simulink model "tv_system_sqabs"  (R2021b)
settings: Solver=VariableStepAuto  StartTime=0.0  StopTime=0  RelTol=1e-3
values from neighbouring files (symbols this model uses):
  gamma1 = 0.005    [main_pixloss.m]
  gamma2 = 1/(1.05*tau2)*(1/gamma1-beta/2)    [main_pixloss.m]
  lambda = 0.012    [main_pixloss.m]
  maxIter = 500    [main_pixloss.m]
undefined symbols (not defined in the file or in its folder): cols, gray, rows
libraries: visionsources x3, visionstatistics x2
settings Model: Creator=abeshu  LastModifiedBy=shu_abe

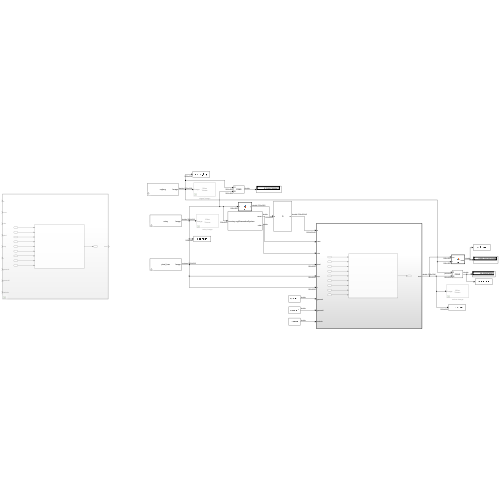
[thumbnail: Simulink's stored preview of the top-level diagram]
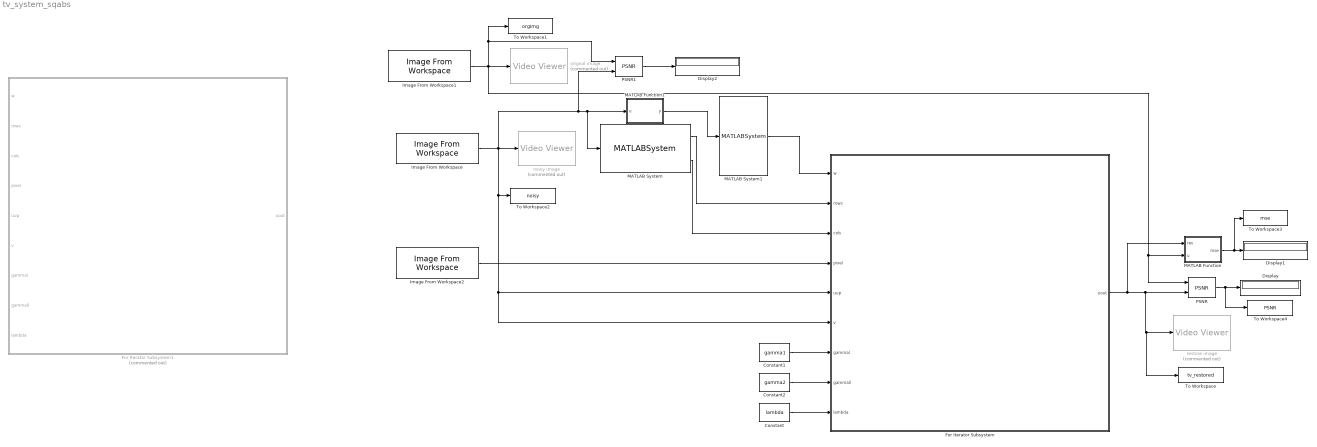
== system tv_system_sqabs ==
  Constant : Constant  Value=lambda
  Constant1 : Constant  Value=gamma1
  Constant2 : Constant  Value=gamma2
  Display : Display
  Display1 : Display
  Display2 : Display
  For Iterator Subsystem : Subsystem  TreatAsAtomicUnit=on
  For Iterator Subsystem1 : Subsystem  Commented=on  TreatAsAtomicUnit=on
  Image From Workspace : visionsources/Image From Workspace  Tag=vipblks_nd  ImageValue=noisy  Ts=inf  imagePorts=One multidimensional signal  OutPortLabels=R|G|B  ImageDataType=Inherit from 'Value'  Signed=on  WordLength=16  sdImageDataType=sfix(16)  FractionLengthMode=User-defined  FractionLength=15
      settings: SourceProductBaseCode=VP
  Image From Workspace1 : visionsources/Image From Workspace  Tag=vipblks_nd  ImageValue=orgImg  Ts=inf  imagePorts=One multidimensional signal  OutPortLabels=R|G|B  ImageDataType=Inherit from 'Value'  Signed=on  WordLength=16  sdImageDataType=sfix(16)  FractionLengthMode=User-defined  FractionLength=15
      settings: SourceProductBaseCode=VP
  Image From Workspace2 : visionsources/Image From Workspace  Tag=vipblks_nd  ImageValue=pixel_loss  Ts=inf  imagePorts=One multidimensional signal  OutPortLabels=R|G|B  ImageDataType=Inherit from 'Value'  Signed=on  WordLength=16  sdImageDataType=sfix(16)  FractionLengthMode=User-defined  FractionLength=15
      settings: SourceProductBaseCode=VP
  MATLAB Function : MATLAB Function  TreatAsAtomicUnit=on
  MATLAB Function1 : MATLAB Function  TreatAsAtomicUnit=on
  MATLAB System : MATLABSystem  System=regObsevationSystem  SimulateUsing=Code generation
      mask Type: regObsevationSystem
      mask Display:
      | disp('regObsevationSystem');
      | port_label('input',1,'imnoisy');
      | port_label('output',1,'rows');
      | port_label('output',2,'colw');
  MATLAB System1 : MATLABSystem  System=dBlockSystem  SimulateUsing=Code generation
      mask Type: dBlockSystem
      mask Display:
      | disp('D');
      | port_label('input',1,'z');
      | port_label('output',1,'w');
  PSNR : visionstatistics/PSNR
      settings: SourceProductBaseCode=VP
  PSNR1 : visionstatistics/PSNR
      settings: SourceProductBaseCode=VP
  To Workspace : ToWorkspace  VariableName=tv_restored  SaveFormat=Structure  SampleTime=-1
      settings: Save2DSignal=2-D array (concatenate along first dimension)
  To Workspace1 : ToWorkspace  VariableName=orgImg  SaveFormat=Structure  SampleTime=-1
      settings: Save2DSignal=2-D array (concatenate along first dimension)
  To Workspace2 : ToWorkspace  VariableName=noisy  SaveFormat=Structure  SampleTime=-1
      settings: Save2DSignal=2-D array (concatenate along first dimension)
  To Workspace3 : ToWorkspace  VariableName=mse  SaveFormat=Structure  SampleTime=-1
      settings: Save2DSignal=2-D array (concatenate along first dimension)
  To Workspace4 : ToWorkspace  VariableName=PSNR  SaveFormat=Structure  SampleTime=-1
      settings: Save2DSignal=2-D array (concatenate along first dimension)
  noisy image : VideoViewer  Commented=on  FigPos=[211 982 368 339]
  orignal image : VideoViewer  Commented=on  FigPos=[20 546 468 269]
  restore image : VideoViewer  Commented=on  colormapValue=gray(256)  FigPos=[260 843 480 394]
  wires:
  Image From Workspace/1 -> For Iterator Subsystem/6(v), For Iterator Subsystem/5(uup), To Workspace2/1, PSNR1/2, MATLAB System/1, MATLAB Function1/1(u), noisy image/1
  Image From Workspace1/1 -> PSNR1/1, To Workspace1/1, PSNR/1, MATLAB Function/2(u), orignal image/1
  Image From Workspace2/1 -> For Iterator Subsystem/4(pixel)
  MATLAB System/1 -> For Iterator Subsystem/2(rows)
  MATLAB System/2 -> For Iterator Subsystem/3(cols)
  MATLAB Function1/1(y) -> MATLAB System1/1
  Constant1/1 -> For Iterator Subsystem/7(gammal)
  Constant2/1 -> For Iterator Subsystem/8(gammall)
  Constant/1 -> For Iterator Subsystem/9(lambda)
  MATLAB System1/1 -> For Iterator Subsystem/1(w)
  For Iterator Subsystem/1(uout) -> MATLAB Function/1(res), To Workspace/1, restore image/1, PSNR/2
  PSNR/1 -> To Workspace4/1, Display/1
  MATLAB Function/1(mse) -> To Workspace3/1, Display1/1
  PSNR1/1 -> Display2/1

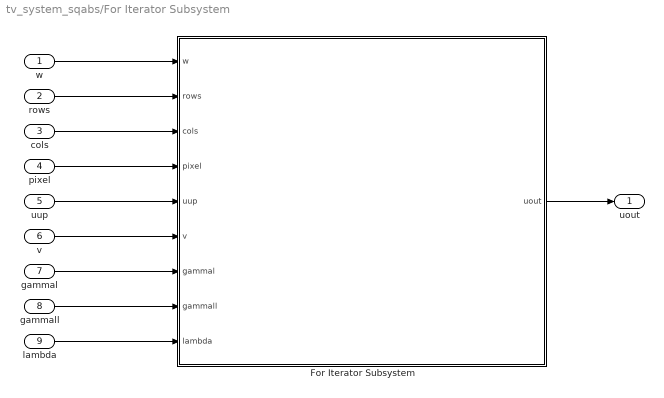
== system tv_system_sqabs/For Iterator Subsystem ==
  w : Inport
  rows : Inport  Port=2
  cols : Inport  Port=3
  pixel : Inport  Port=4
  uup : Inport  Port=5
  v : Inport  Port=6
  gammal : Inport  Port=7
  gammall : Inport  Port=8
  lambda : Inport  Port=9
  For Iterator Subsystem : Subsystem  TreatAsAtomicUnit=on
  uout : Outport
  wires:
  For Iterator Subsystem/1(uout) -> uout/1
  w/1 -> For Iterator Subsystem/1(w)
  rows/1 -> For Iterator Subsystem/2(rows)
  cols/1 -> For Iterator Subsystem/3(cols)
  pixel/1 -> For Iterator Subsystem/4(pixel)
  uup/1 -> For Iterator Subsystem/5(uup)
  v/1 -> For Iterator Subsystem/6(v)
  gammal/1 -> For Iterator Subsystem/7(gammal)
  gammall/1 -> For Iterator Subsystem/8(gammall)
  lambda/1 -> For Iterator Subsystem/9(lambda)

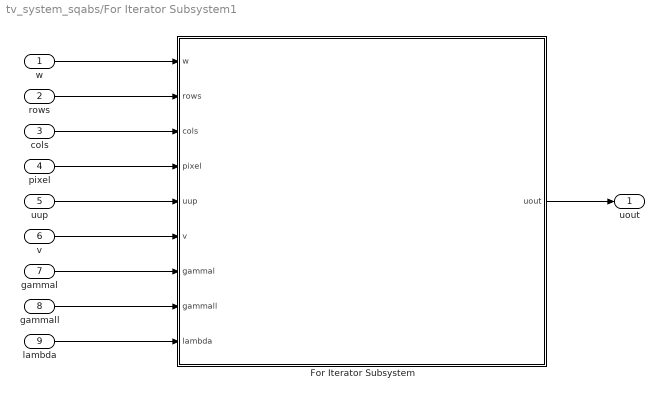
== system tv_system_sqabs/For Iterator Subsystem1 ==
  w : Inport
  rows : Inport  Port=2
  cols : Inport  Port=3
  pixel : Inport  Port=4
  uup : Inport  Port=5
  v : Inport  Port=6
  gammal : Inport  Port=7
  gammall : Inport  Port=8
  lambda : Inport  Port=9
  For Iterator Subsystem : Subsystem  TreatAsAtomicUnit=on
  uout : Outport
  wires:
  For Iterator Subsystem/1(uout) -> uout/1
  w/1 -> For Iterator Subsystem/1(w)
  rows/1 -> For Iterator Subsystem/2(rows)
  cols/1 -> For Iterator Subsystem/3(cols)
  pixel/1 -> For Iterator Subsystem/4(pixel)
  uup/1 -> For Iterator Subsystem/5(uup)
  v/1 -> For Iterator Subsystem/6(v)
  gammal/1 -> For Iterator Subsystem/7(gammal)
  gammall/1 -> For Iterator Subsystem/8(gammall)
  lambda/1 -> For Iterator Subsystem/9(lambda)

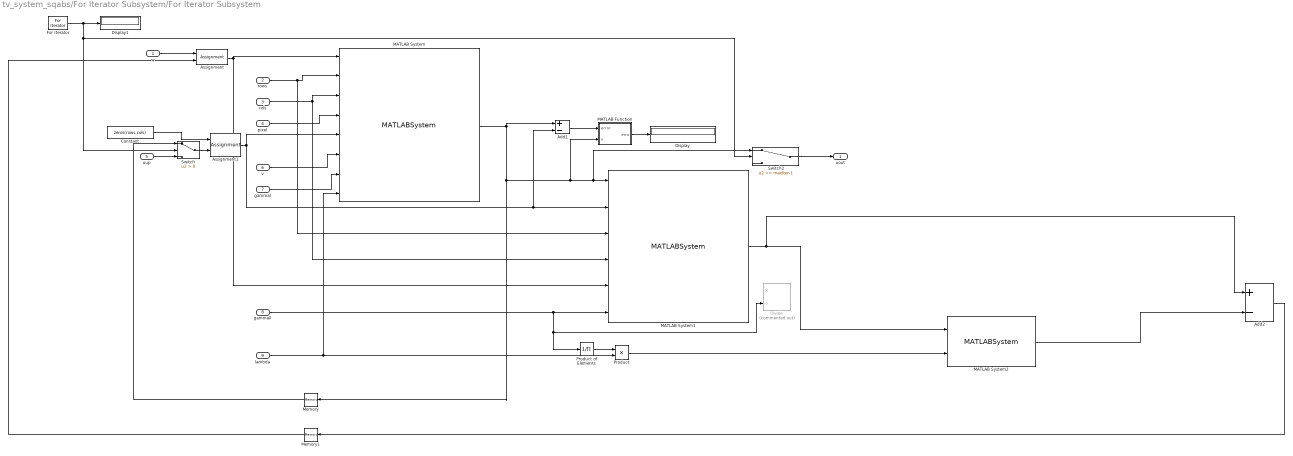
== system tv_system_sqabs/For Iterator Subsystem/For Iterator Subsystem ==
  w : Inport
  rows : Inport  Port=2
  cols : Inport  Port=3
  pixel : Inport  Port=4
  uup : Inport  Port=5
  v : Inport  Port=6
  gammal : Inport  Port=7
  gammall : Inport  Port=8
  lambda : Inport  Port=9
  Add1 : Sum  Inputs=+-
  Add2 : Sum  Inputs=+-
  Assignment : Assignment  NumberOfDimensions=3  DiagnosticForDimensions=Warning  IndexOptions=Assign all,Assign all,Assign all  Indices=1,1,1  OutputSizes=1,1,1
  Assignment1 : Assignment  NumberOfDimensions=2  DiagnosticForDimensions=Warning  IndexOptions=Assign all,Assign all  Indices=1,1  OutputSizes=1,1
  Constant : Constant  Value=zeros(rows,cols)
  Display : Display
  Display1 : Display
  Divide : Product  Commented=on  Inputs=*/
  For Iterator : ForIterator  IterationLimit=maxIter  IndexMode=Zero-based  IterationVariableDataType=double
  MATLAB Function : MATLAB Function  TreatAsAtomicUnit=on
  MATLAB System : MATLABSystem  System=updateuSystem  SimulateUsing=Code generation
      mask Type: updateuSystem
      mask Display:
      | disp('updateuSystem');
      | port_label('input',1,'w');
      | port_label('input',2,'rows');
      | port_label('input',3,'cols');
      | port_label('input',4,'pixel');
      | port_label('input',5,'uup');
      | port_label('input',6,'v');
      | port_label('input',7,'gamma1');
      | port_label('input',8,'lambda');
      | port_label('output',1,'u');
  MATLAB System1 : MATLABSystem  System=updatewSystem  SimulateUsing=Code generation
      mask Type: updatewSystem
      mask Display:
      | disp('updatewSystem');
      | port_label('input',1,'u');
      | port_label('input',2,'upre');
      | port_label('input',3,'rows');
      | port_label('input',4,'cols');
      | port_label('input',5,'w');
      | port_label('input',6,'gamma2');
      | port_label('output',1,'w_tilde');
  MATLAB System2 : MATLABSystem  System=SoftThrSystem  SimulateUsing=Code generation
      mask Type: SoftThrSystem
      mask Display:
      | disp('SoftThrSystem');
      | port_label('input',1,'x');
      | port_label('input',2,'lambda');
      | port_label('output',1,'y');
  Memory : Memory  InheritSampleTime=on
  Memory1 : Memory  InheritSampleTime=on
  Product : Product
  Product of Elements : Product  Inputs=/
  Switch : Switch  Criteria=u2 > Threshold
  Switch2 : Switch  Threshold=maxIter-1
  uout : Outport
  wires:
  w/1 -> Assignment/1
  Assignment/1 -> MATLAB System/1, MATLAB System1/5
  rows/1 -> MATLAB System/2, MATLAB System1/3
  cols/1 -> MATLAB System1/4, MATLAB System/3
  pixel/1 -> MATLAB System/4
  Constant/1 -> Assignment1/1
  Switch/1 -> Assignment1/2
  uup/1 -> Switch/3
  Assignment1/1 -> Add1/2, MATLAB System1/2, MATLAB System/5
  v/1 -> MATLAB System/6
  gammal/1 -> MATLAB System/7
  For Iterator/1 -> Switch/2, Switch2/2, Display1/1
  MATLAB System/1 -> Add1/1, Switch2/1, MATLAB System1/1, MATLAB Function/2(u), Memory/1
  Add1/1 -> MATLAB Function/1(error)
  MATLAB Function/1(erro) -> Display/1
  gammall/1 -> Product of Elements/1, Divide/2, MATLAB System1/6
  MATLAB System1/1 -> MATLAB System2/1, Add2/1
  Product of Elements/1 -> Product/1
  lambda/1 -> MATLAB System/8, Product/2
  Product/1 -> MATLAB System2/2
  Memory/1 -> Switch/1
  Add2/1 -> Memory1/1
  MATLAB System2/1 -> Add2/2
  Memory1/1 -> Assignment/2
  Switch2/1 -> uout/1

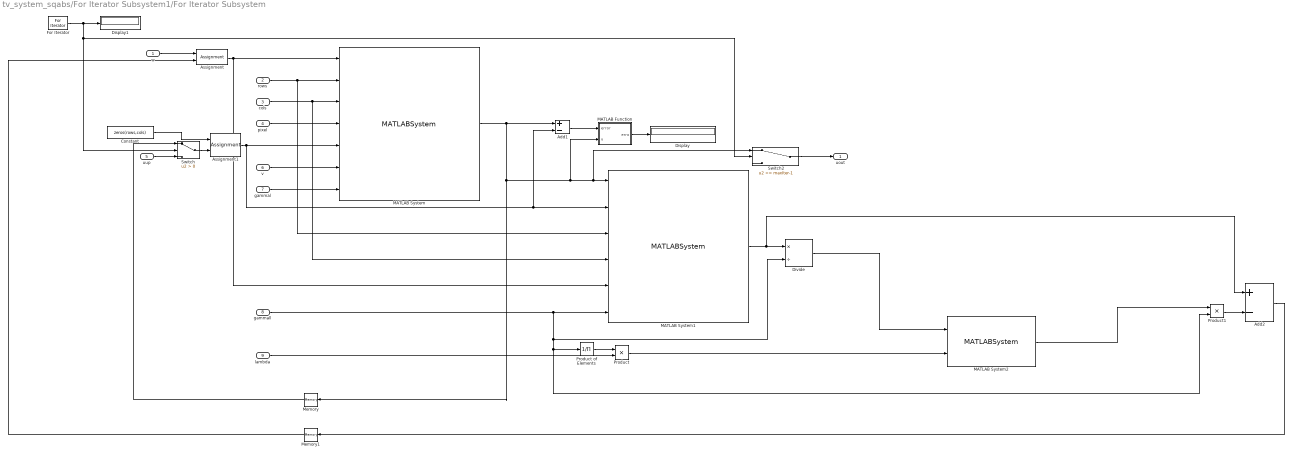
== system tv_system_sqabs/For Iterator Subsystem1/For Iterator Subsystem ==
  w : Inport
  rows : Inport  Port=2
  cols : Inport  Port=3
  pixel : Inport  Port=4
  uup : Inport  Port=5
  v : Inport  Port=6
  gammal : Inport  Port=7
  gammall : Inport  Port=8
  lambda : Inport  Port=9
  Add1 : Sum  Inputs=+-
  Add2 : Sum  Inputs=+-
  Assignment : Assignment  NumberOfDimensions=3  DiagnosticForDimensions=Warning  IndexOptions=Assign all,Assign all,Assign all  Indices=1,1,1  OutputSizes=1,1,1
  Assignment1 : Assignment  NumberOfDimensions=2  DiagnosticForDimensions=Warning  IndexOptions=Assign all,Assign all  Indices=1,1  OutputSizes=1,1
  Constant : Constant  Value=zeros(rows,cols)
  Display : Display
  Display1 : Display
  Divide : Product  Inputs=*/
  For Iterator : ForIterator  IterationLimit=maxIter  IndexMode=Zero-based  IterationVariableDataType=double
  MATLAB Function : MATLAB Function  TreatAsAtomicUnit=on
  MATLAB System : MATLABSystem  System=updateuSystem  SimulateUsing=Code generation
      mask Type: updateuSystem
      mask Display:
      | disp('updateuSystem');
      | port_label('input',1,'w');
      | port_label('input',2,'rows');
      | port_label('input',3,'cols');
      | port_label('input',4,'pixel');
      | port_label('input',5,'uup');
      | port_label('input',6,'v');
      | port_label('input',7,'gamma1');
      | port_label('output',1,'u');
  MATLAB System1 : MATLABSystem  System=updatewSystem  SimulateUsing=Code generation
      mask Type: updatewSystem
      mask Display:
      | disp('updatewSystem');
      | port_label('input',1,'u');
      | port_label('input',2,'upre');
      | port_label('input',3,'rows');
      | port_label('input',4,'cols');
      | port_label('input',5,'w');
      | port_label('input',6,'gamma2');
      | port_label('output',1,'w_tilde');
  MATLAB System2 : MATLABSystem  System=SoftThrSystem  SimulateUsing=Code generation
      mask Type: SoftThrSystem
      mask Display:
      | disp('SoftThrSystem');
      | port_label('input',1,'x');
      | port_label('input',2,'lambda');
      | port_label('output',1,'y');
  Memory : Memory  InheritSampleTime=on
  Memory1 : Memory  InheritSampleTime=on
  Product : Product
  Product of Elements : Product  Inputs=/
  Product1 : Product
  Switch : Switch  Criteria=u2 > Threshold
  Switch2 : Switch  Threshold=maxIter-1
  uout : Outport
  wires:
  w/1 -> Assignment/1
  Assignment/1 -> MATLAB System/1, MATLAB System1/5
  rows/1 -> MATLAB System/2, MATLAB System1/3
  cols/1 -> MATLAB System1/4, MATLAB System/3
  pixel/1 -> MATLAB System/4
  Constant/1 -> Assignment1/1
  Switch/1 -> Assignment1/2
  uup/1 -> Switch/3
  Assignment1/1 -> Add1/2, MATLAB System1/2, MATLAB System/5
  v/1 -> MATLAB System/6
  gammal/1 -> MATLAB System/7
  For Iterator/1 -> Switch/2, Switch2/2, Display1/1
  MATLAB System/1 -> Switch2/1, MATLAB System1/1, MATLAB Function/2(u), Memory/1, Add1/1
  Add1/1 -> MATLAB Function/1(error)
  MATLAB Function/1(erro) -> Display/1
  gammall/1 -> Product1/2, Product of Elements/1, Divide/2, MATLAB System1/6
  MATLAB System1/1 -> Add2/1, Divide/1
  Divide/1 -> MATLAB System2/1
  Product of Elements/1 -> Product/1
  lambda/1 -> Product/2
  Product/1 -> MATLAB System2/2
  Memory/1 -> Switch/1
  MATLAB System2/1 -> Product1/1
  Add2/1 -> Memory1/1
  Product1/1 -> Add2/2
  Memory1/1 -> Assignment/2
  Switch2/1 -> uout/1

== matlab function tv_system_sqabs/For Iterator Subsystem1/For Iterator Subsystem/MATLAB Function ==
  data: error input; u input; erro output
function erro = fcn(error,u)

erro = norm(error(:),2) / norm(u(:),2);

== matlab function tv_system_sqabs/For Iterator Subsystem/For Iterator Subsystem/MATLAB Function ==
  data: error input; u input; erro output
function erro = fcn(error,u)

erro = norm(error(:),2) / norm(u(:),2);

== matlab function tv_system_sqabs/MATLAB Function ==
  data: res input; u input; mse output
function mse = fcn(res,u)

mse = immse(u,res);

== matlab function tv_system_sqabs/MATLAB Function1 ==
  data: u input; y output
function y = fcn(u)

y = zeros(size(u));
